simulink model "shell1"  (R2016b)
settings: Solver=VariableStepAuto  StartTime=0.0  StopTime=5  RelTol=1e-3
libraries: cstblocks x2
settings Model: Creator=m184410  LastModifiedBy=m181524

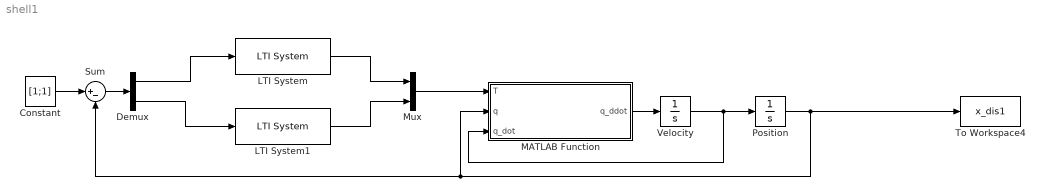
== system shell1 ==
  Constant : Constant  Value=[1;1]
  Demux : Demux  Outputs=2
  LTI System : cstblocks/LTI System  sys=KGc1  IC=[]
  LTI System1 : cstblocks/LTI System  sys=KGc2  IC=[]
  MATLAB Function : MATLAB Function  TreatAsAtomicUnit=on
  Mux : Mux  Inputs=2
  Position : Integrator  InitialCondition=[0;0]
  Sum : Sum  Inputs=|+-
  To Workspace4 : ToWorkspace  VariableName=x_dis1  SaveFormat=Timeseries  SampleTime=-1
  Velocity : Integrator  InitialCondition=[0;0]
  wires:
  MATLAB Function/1(q_ddot) -> Velocity/1
  Velocity/1 -> MATLAB Function/3(q_dot), Position/1
  Position/1 -> To Workspace4/1, Sum/2, MATLAB Function/2(q)
  Mux/1 -> MATLAB Function/1(T)
  LTI System1/1 -> Mux/2
  LTI System/1 -> Mux/1
  Demux/1 -> LTI System/1
  Demux/2 -> LTI System1/1
  Sum/1 -> Demux/1
  Constant/1 -> Sum/1

== matlab function shell1/MATLAB Function ==
  data: T input; q input; q_dot input; q_ddot output
function q_ddot = nonlinear_model(T,q,q_dot)

m1 = 3.31;
m2 = 0.116;
m3 = 0.16;
fd1 = 2.0;
fd2 = 0.5;

M = [ m1+2*m3*cos(q(2)) , m2+m3*cos(q(2)) ;
      m2+m3*cos(q(2)) , m2 ];
Vm = [ -m3*sin(q(2))*q_dot(2) , -m3*sin(q(2))*(q_dot(1)+q_dot(2)) ;
       m3*sin(q(2))*q_dot(1) , 0];
Ft = [fd1 , 0 ; 0 , fd2 ];

q_ddot = M^(-1) * (T - Vm * q_dot - Ft * q_dot);

end
